simulink model "ssc_lithium_battery_1CellMultiplied"  (Simulink 7.6)
settings: Solver=ode15s  StartTime=0.0  StopTime=40000  MaxStep=600  RelTol=1e-3
PreLoadFcn:
  | ssc_lithium_battery_80Cells_ini
values from neighbouring files (symbols this model uses):
  BatteryParams = struct()    [ssc_lithium_battery_80Cells_ini.m]
  numCells = 80    [ssc_lithium_battery_80Cells_ini.m]
undefined symbols (not defined in the file or in its folder): sigbuilder_block
libraries: fl_lib x14, nesl_utility x4, LiBatteryBlocks x1
settings Model: Creator=rjackey  LastModifiedBy=rjackey
settings DebuggingCC: FcnCallInpInsideContextMsg=Enable All
settings GRTTargetCC: CombineOutputUpdateFcns=on

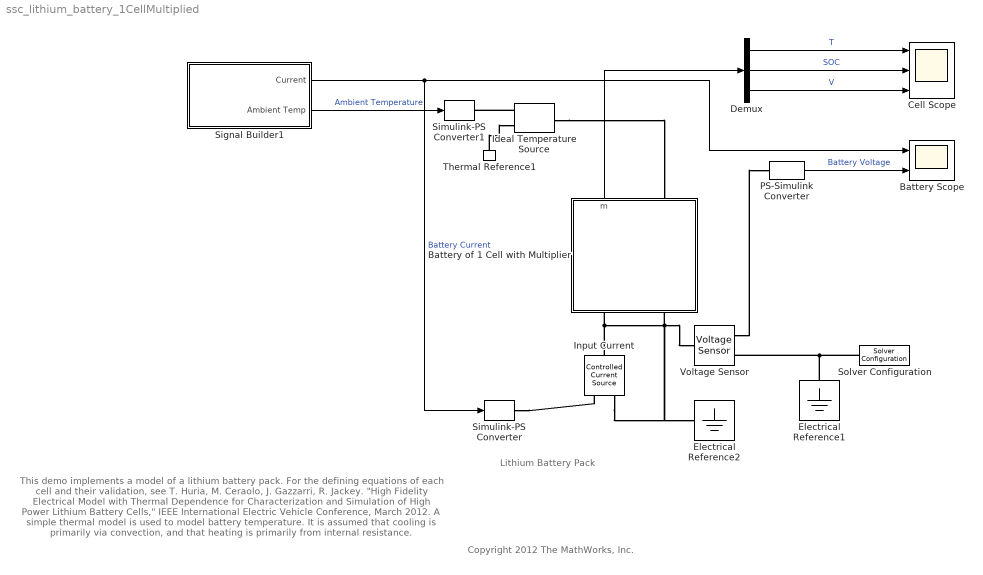
== system ssc_lithium_battery_1CellMultiplied ==
  note: Lithium Battery Pack
  note: This demo implements a model of a lithium battery pack. For the defining equations of each cell and their validation, see T. Huria, M. Ceraolo,
      | J. Gazzarri, R. Jackey. "High Fidelity Electrical Model with Thermal Dependence for Characterization and Simulation of High Power Lithium
      | Battery Cells," IEEE International Electric Vehicle Conference, March 2012. A simple thermal model is used to model battery temperature. It is
      | assumed that cooling is primarily via convection, and that heating is primarily from internal resistance.
  note: Copyright 2012 The MathWorks, Inc.
  Battery Scope : Scope  NumInputPorts=2
      settings: TimeRange=40000  YMin=-30~250  YMax=10~350
  Battery of 1 Cell with Multiplier : Subsystem
  Cell Scope : Scope  NumInputPorts=3
      settings: TimeRange=40000  YMin=20~0~3  YMax=23.5~1~4.5
  Demux : Demux  Outputs=3
  Electrical Reference1 : fl_lib/Electrical/Electrical Elements/Electrical Reference  DialogController=NetworkEngine.DynNeDlgSource  SystemSampleTime=-1  i_Log=off  LocalVarNames=|i  LocalVarDescs=|i  LocalVarLogging=0
  Electrical Reference2 : fl_lib/Electrical/Electrical Elements/Electrical Reference  DialogController=NetworkEngine.DynNeDlgSource  SystemSampleTime=-1  i_Log=off  LocalVarNames=|i  LocalVarDescs=|i  LocalVarLogging=0
  Ideal Temperature Source : fl_lib/Thermal/Thermal Sources/Ideal Temperature Source  DialogController=NetworkEngine.DynNeDlgSource  SystemSampleTime=-1  Q_Log=off  T_Log=off  LocalVarNames=|heat_flow|T_differential  LocalVarDescs=|Heat flow rate through the source (J/s)|Temperature differential across the source (K)  LocalVarLogging=[0 0]
  Input Current : fl_lib/Electrical/Electrical Sources/Controlled Current Source  DialogController=NetworkEngine.DynNeDlgSource  SystemSampleTime=-1  i_Log=off  v_Log=off  LocalVarNames=|current|voltage|power  LocalVarDescs=|Current (A)|Voltage (V)|Power (W)  LocalVarLogging=[0 0 0]
  PS-Simulink Converter : nesl_utility/PS-Simulink Converter  DialogController=NetworkEngine.DynNeUtilDlgSource  SystemSampleTime=-1  PhysicalDomain=network_engine_domain  LeftPortType=input  RightPortType=output  SubClassName=ps_output  Unit=V  AffineConversion=off
  Signal Builder1 : Subsystem  Tag=STV Subsys  LoadFcn=sigbuilder_block('load');  StartFcn=sigbuilder_block('start');  StopFcn=sigbuilder_block('stop');  ClipboardFcn=sigbuilder_block('clipboard');  mask(Sigbuilder block){}
      mask help: Simulink:masks:SigbuilderBlock_MD
      mask init:
      | if ~strcmp(get_param(bdroot(gcbh),'SimulationStatus'),'stopped') tuvar = sigbuilder_block('maskInit'); end
      settings: CopyFcn=sigbuilder_block('copy');  DeleteFcn=sigbuilder_block('delete');  ModelCloseFcn=sigbuilder_block('modelClose');  PreSaveFcn=sigbuilder_block('preSave');  NameChangeFcn=sigbuilder_block('namechange');  OpenFcn=sigbuilder_block('open',[28.5 123.75 755.25 399.75 ]);  CloseFcn=sigbuilder_block('close');
      mask Display: plot(0,0,100,100,[10,10,40,40,10],[80,20,20,80,80],[40,10],[50,50], [40,27,10],[65,72,56],[40,25,25,10],[28,28,43,43]);
  Simulink-PS Converter : nesl_utility/Simulink-PS Converter  DialogController=NetworkEngine.DynNeUtilDlgSource  SystemSampleTime=-1  PhysicalDomain=network_engine_domain  LeftPortType=input  RightPortType=output  SubClassName=ps_input  Unit=A  AffineConversion=on  InputFilterTimeConstant=.001  UdotUserProvided=0
  Simulink-PS Converter1 : nesl_utility/Simulink-PS Converter  DialogController=NetworkEngine.DynNeUtilDlgSource  SystemSampleTime=-1  PhysicalDomain=network_engine_domain  LeftPortType=input  RightPortType=output  SubClassName=ps_input  Unit=C  AffineConversion=on  InputFilterTimeConstant=.001  UdotUserProvided=0
  Solver Configuration : nesl_utility/Solver Configuration  DialogController=NetworkEngine.DynNeUtilDlgSource  SystemSampleTime=-1  PhysicalDomain=network_engine_domain  LeftPortType=input  RightPortType=generic  SubClassName=solver  Accelerate=off  Profile=off  ResidualTolerance=1e-9  MaxNonlinIter=3  MaxModeIter=2  DoFixedCost=off  UseLocalSampling=off  DoDC=off  LinearAlgebra=Sparse  LocalSolverSampleTime=.001  LocalSolverChoice=NE_BACKWARD_EULER_ADVANCER  UseLocalSolver=off
  Thermal Reference1 : fl_lib/Thermal/Thermal Elements/Thermal Reference  DialogController=NetworkEngine.DynNeDlgSource  SystemSampleTime=-1  Q_Log=off  LocalVarNames=|Q  LocalVarDescs=|Q  LocalVarLogging=[]
  Voltage Sensor : fl_lib/Electrical/Electrical Sensors/Voltage Sensor  DialogController=NetworkEngine.DynNeDlgSource  SystemSampleTime=-1  i1_Log=off  v1_Log=off  LocalVarNames=|i1|v1  LocalVarDescs=|i1|v1  LocalVarLogging=[0 0]
  wires:
  Demux/2 -> Cell Scope/2  "SOC"
  Demux/3 -> Cell Scope/3  "V"
  PS-Simulink Converter/1 -> Battery Scope/2  "Battery Voltage"
  Battery of 1 Cell with Multiplier/1(m) -> Demux/1
  Signal Builder1/1(Current) -> Simulink-PS Converter/1, Battery Scope/1  "Battery Current"
  Signal Builder1/2(Ambient Temp) -> Simulink-PS Converter1/1  "Ambient Temperature"
  Demux/1 -> Cell Scope/1  "T"
  connections:
  Ideal Temperature Source/RConn1 -- Simulink-PS Converter1/RConn1
  Thermal Reference1/LConn1 -- Ideal Temperature Source/RConn2
  Simulink-PS Converter/RConn1 -- Input Current/RConn1
  Electrical Reference1/LConn1 -- Voltage Sensor/RConn2 -- Solver Configuration/RConn1
  Battery of 1 Cell with Multiplier/LConn1 -- Voltage Sensor/LConn1 -- Input Current/LConn1
  Battery of 1 Cell with Multiplier/LConn2 -- Input Current/RConn2 -- Electrical Reference2/LConn1
  Voltage Sensor/RConn1 -- PS-Simulink Converter/LConn1
  Ideal Temperature Source/LConn1 -- Battery of 1 Cell with Multiplier/RConn1

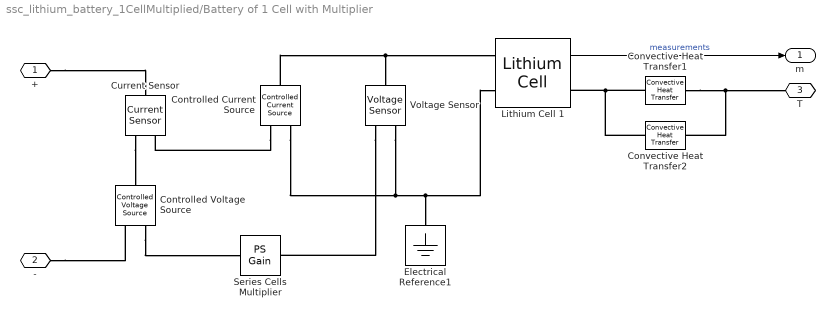
== system ssc_lithium_battery_1CellMultiplied/Battery of 1 Cell with Multiplier ==
  Controlled Current Source : fl_lib/Electrical/Electrical Sources/Controlled Current Source  DialogController=NetworkEngine.DynNeDlgSource  SystemSampleTime=-1  i_Log=off  v_Log=off  LocalVarNames=|i|v  LocalVarDescs=|i|v  LocalVarLogging=[0 0]
  Controlled Voltage Source : fl_lib/Electrical/Electrical Sources/Controlled Voltage Source  DialogController=NetworkEngine.DynNeDlgSource  SystemSampleTime=-1  i_Log=off  v_Log=off  LocalVarNames=|i|v  LocalVarDescs=|i|v  LocalVarLogging=[0 0]
  Convective Heat Transfer1 : fl_lib/Thermal/Thermal Elements/Convective Heat Transfer  DialogController=NetworkEngine.DynNeDlgSource  SystemSampleTime=-1  area=cell_area m^2  heat_tr_coeff=h_conv_end W/(m^2 * K)  Q_Log=off  T_Log=off  LocalVarNames=|heat_flow|temperature_diff  LocalVarDescs=|Heat flow (J/s)|Temperature difference (K)  LocalVarLogging=[0 0]
  Convective Heat Transfer2 : fl_lib/Thermal/Thermal Elements/Convective Heat Transfer  DialogController=NetworkEngine.DynNeDlgSource  SystemSampleTime=-1  area=cell_area m^2  heat_tr_coeff=h_conv_end W/(m^2 * K)  Q_Log=off  T_Log=off  LocalVarNames=|heat_flow|temperature_diff  LocalVarDescs=|Heat flow (J/s)|Temperature difference (K)  LocalVarLogging=[0 0]
  Current Sensor : fl_lib/Electrical/Electrical Sensors/Current Sensor  DialogController=NetworkEngine.DynNeDlgSource  SystemSampleTime=-1  i1_Log=off  v1_Log=off  LocalVarNames=|i1|v1  LocalVarDescs=|i1|v1  LocalVarLogging=[0 0]
  Electrical Reference1 : fl_lib/Electrical/Electrical Elements/Electrical Reference  DialogController=NetworkEngine.DynNeDlgSource  SystemSampleTime=-1  i_Log=off  LocalVarNames=|i  LocalVarDescs=|i  LocalVarLogging=[]
  Lithium Cell 1 : LiBatteryBlocks/Lithium Cell  SystemSampleTime=-1  Battery=BatteryParams(1)
      settings: AttributesFormatString=%<Battery>
  Series Cells Multiplier : fl_lib/Physical Signals/Functions/PS Gain  DialogController=NetworkEngine.DynNeDlgSource  SystemSampleTime=-1  gain=numCells  LocalVarLogging=[]
  Voltage Sensor : fl_lib/Electrical/Electrical Sensors/Voltage Sensor  DialogController=NetworkEngine.DynNeDlgSource  SystemSampleTime=-1  i1_Log=off  v1_Log=off  LocalVarNames=|i1|v1  LocalVarDescs=|i1|v1  LocalVarLogging=[0 0]
  + : PMIOPort  Port=1  Side=Left
  - : PMIOPort  Port=2  Side=Left
  T : PMIOPort  Port=3  Side=Right
  m : Outport
  wires:
  Lithium Cell 1/1 -> m/1  "measurements"
  connections:
  Current Sensor/RConn2 -- Controlled Voltage Source/LConn1
  Convective Heat Transfer1/RConn1 -- Lithium Cell 1/RConn1 -- Convective Heat Transfer2/RConn1
  Convective Heat Transfer1/LConn1 -- T/RConn1 -- Convective Heat Transfer2/LConn1
  Controlled Current Source/LConn1 -- Lithium Cell 1/LConn1 -- Voltage Sensor/LConn1
  Controlled Current Source/RConn2 -- Lithium Cell 1/LConn2 -- Electrical Reference1/LConn1 -- Voltage Sensor/RConn2
  Controlled Current Source/RConn1 -- Current Sensor/RConn1
  -/RConn1 -- Controlled Voltage Source/RConn2
  +/RConn1 -- Current Sensor/LConn1
  Controlled Voltage Source/RConn1 -- Series Cells Multiplier/RConn1
  Voltage Sensor/RConn1 -- Series Cells Multiplier/LConn1

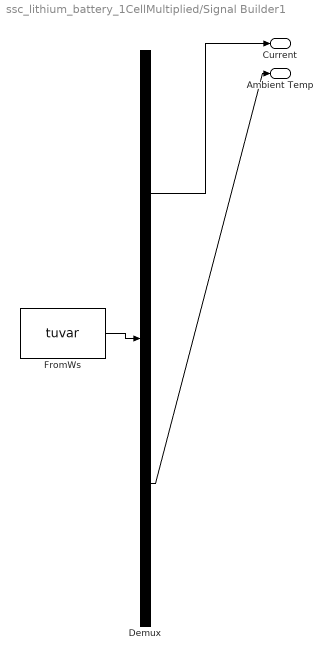
== system ssc_lithium_battery_1CellMultiplied/Signal Builder1 ==
  Demux : Demux  Tag=STV Demux  Outputs=2
  FromWs : FromWorkspace  Tag=STV FromWs  VariableName=tuvar  SampleTime=0  SigBuilderData=DataTag0  VnvData=DataTag1
      SigBuilderData=|
      | common.afterFinalStr = 'Extrapolate'
      | common.sampleTime = 0
      | dataSet(1).timeRange = [0 40000]
      | dataSet(1).name = 'Pulse'
      | dataSet(2).timeRange = [0 40000]
      | dataSet(2).name = 'Constant'
      | sbobj.Name = 'Signal Builder'
      | sbobj.Groups(1).Name = 'Pulse'
      | sbobj.Groups(1).Signals(1).Name = 'Current'
      | sbobj.Groups(1).Signals(1).XData = [0 300 300 1900 1900 3600 3600 3960 3960 7200 7200 7560 7560 10800 10800 11160 11160 14400 14400 14760 14760 18000 18000 18360 18360 21600 21600 21960 21960 25200 25200 25560 25560 28800 28800 29160 29160 32400 32400 32760 32760 36000 36000 36360 36360 40000]
      | sbobj.Groups(1).Signals(1).YData = [0 0 7 7 0 0 -27.625 -27.625 0 0 -27.625 -27.625 0 0 -27.625 -27.625 0 0 -27.625 -27.625 0 0 -27.625 -27.625 0 0 -27.625 -27.625 0 0 -27.625 -27.625 0 0 -27.625 -27.625 0 0 -27.625 -27.625 0 0 -27.625 -27.625 0 0]
      | sbobj.Groups(1).Signals(2).Name = 'Ambient Temp'
      | sbobj.Groups(1).Signals(2).XData = [0 300 2100 3600 3960 7200 7560 10800 11160 14400 14760 18000 18360 21600 21960 25200 25560 28800 29160 32400 32760 36000 36360 40000]
      | sbobj.Groups(1).Signals(2).YData = [20 20 20 20 20 20 20 20 20 20 20 20 20 20 20 20 20 20 20 20 20 20 20 20]
      | sbobj.Groups(1).TimeRange = [0 40000]
      | sbobj.Groups(2).Name = 'Constant'
      | sbobj.Groups(2).Signals(1).Name = 'Current'
      | sbobj.Groups(2).Signals(1).XData = [0 360 360 9100 9100 11800 11800 28200 33800 40000]
      | sbobj.Groups(2).Signals(1).YData = [0 0 -5 -5 0 0 5 5 0 0]
      | sbobj.Groups(2).Signals(2).Name = 'Ambient Temp'
      | sbobj.Groups(2).Signals(2).XData = [0 360 360 9100 9100 11800 11800 28200 33800 40000]
      | sbobj.Groups(2).Signals(2).YData = [20 20.09 20.09 22.275 22.275 22.95 22.95 27.05 28.45 30]
      | sbobj.Groups(2).TimeRange = [0 40000]
  Current : Outport
  Ambient Temp : Outport  Tag=STV Outport  Port=2
  wires:
  Demux/1 -> Current/1
  FromWs/1 -> Demux/1
  Demux/2 -> Ambient Temp/1
